simulink model "various_controller"  (R2023a)
settings: Solver=VariableStepAuto  StartTime=0.0  StopTime=10.0  RelTol=1e-3
settings Model: Creator=USER  LastModifiedBy=USER

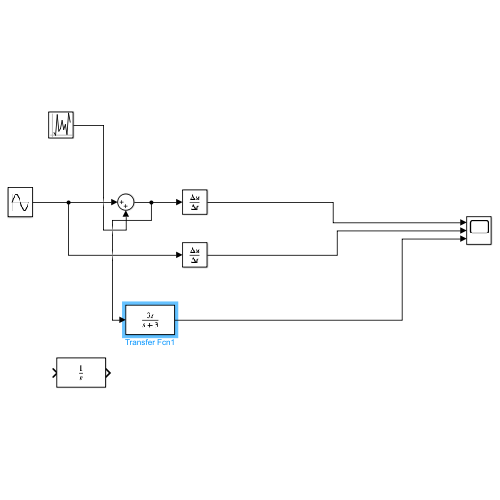
[thumbnail: Simulink's stored preview of the top-level diagram]
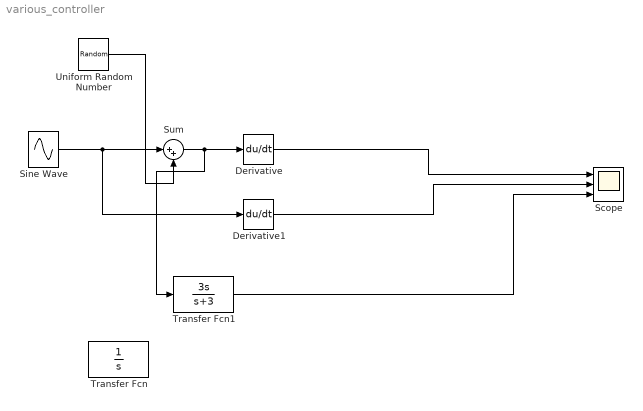
== system various_controller ==
  Derivative : Derivative
  Derivative1 : Derivative
  Scope : Scope  NumInputPorts=3
  Sine Wave : Sin  SampleTime=0
  Sum : Sum  Inputs=|++
  Transfer Fcn : TransferFcn  Denominator=[1 0 ]
  Transfer Fcn1 : TransferFcn  Numerator=[3 0]  Denominator=[1 3]
  Uniform Random Number : UniformRandomNumber  SampleTime=0.1
  wires:
  Derivative/1 -> Scope/1
  Sine Wave/1 -> Derivative1/1, Sum/1
  Uniform Random Number/1 -> Sum/2
  Sum/1 -> Transfer Fcn1/1, Derivative/1
  Derivative1/1 -> Scope/2
  Transfer Fcn1/1 -> Scope/3
